simulink model "internal_cluster_fault"  (R2024b)
settings: Solver=VariableStepAuto  StartTime=0.0  StopTime=120  RelTol=1e-3
undefined symbols (not defined in the file): Ion, Lithium
libraries: spsIGBTDiodeLib x12, spsSeriesRLCBranchLib x4, spsBatteryLib x3, sps_lib x1
settings Model: Creator=Ranbir  LastModifiedBy=Ranbir

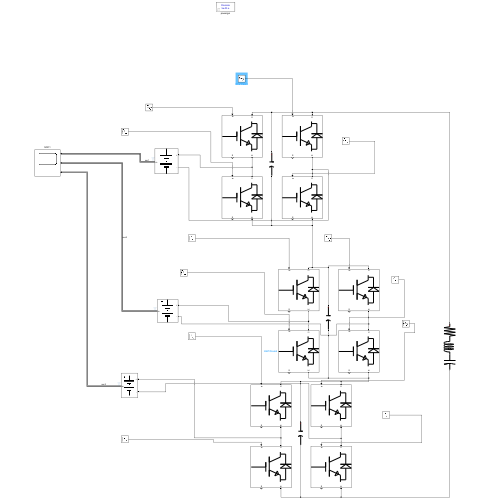
[thumbnail: Simulink's stored preview of the top-level diagram]
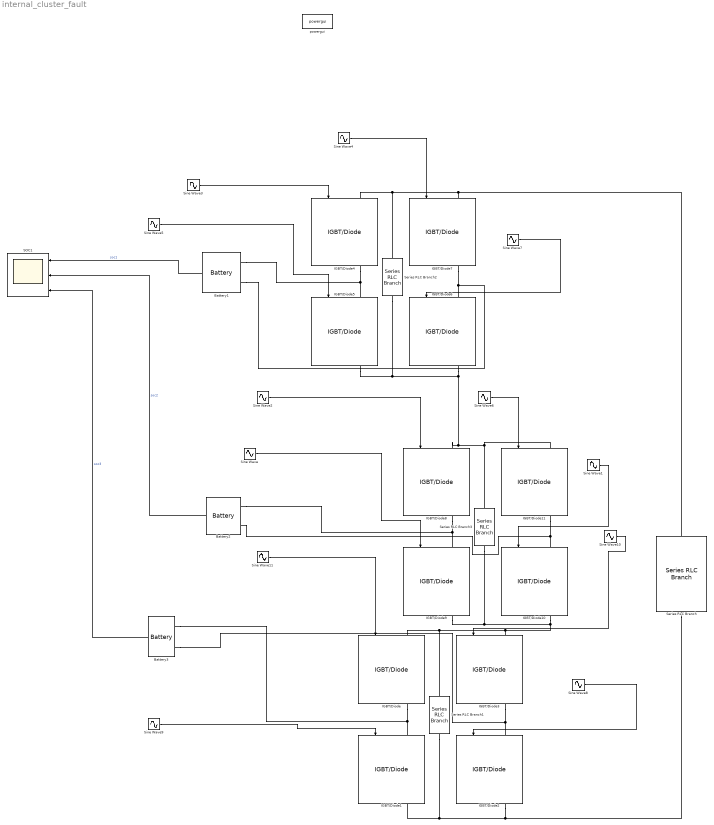
== system internal_cluster_fault ==
  Battery1 : spsBatteryLib/Battery  BatType=Lithium-Ion  NomV=7.2  NomQ=5.4  SOC=75  Batt_Tr=30  PresetModel=on  MaxQ=5.4  MinV=5.4  FullV=8.3807  Dis_rate=2.3478  R=0.013333  Normal_OP=4.8835  expZone="[7.7788      0.2653]"
  Battery2 : spsBatteryLib/Battery  BatType=Lithium-Ion  NomV=7.2  NomQ=5.4  SOC=95  Batt_Tr=30  PresetModel=on  MaxQ=5.4  MinV=5.4  FullV=8.3807  Dis_rate=2.3478  R=0.013333  Normal_OP=4.8835  expZone="[7.7788      0.2653]"
  Battery3 : spsBatteryLib/Battery  BatType=Lithium-Ion  NomV=7.2  NomQ=5.4  SOC=90  Batt_Tr=30  PresetModel=on  MaxQ=5.4  MinV=5.4  FullV=8.3807  Dis_rate=2.3478  R=0.013333  Normal_OP=4.8835  expZone="[7.7788      0.2653]"
  IGBT/Diode{,1..11} (12 alike) : spsIGBTDiodeLib/IGBT//Diode  Ron=1e-3  Rs=1e5  Cs=inf  Measurements=on
  SOC1 : Scope  NumInputPorts=3
  Series RLC Branch : spsSeriesRLCBranchLib/Series RLC Branch  LConnTagsString=__new0  RConnTagsString=__new0  BranchType=RLC  Resistance=1  Inductance=1e-3  SetiL0=off  InitialCurrent=0  Capacitance=1e-6  Setx0=off  InitialVoltage=0  Measurements=None
  Series RLC Branch1 : spsSeriesRLCBranchLib/Series RLC Branch  LConnTagsString=__new0  RConnTagsString=__new0  BranchType=C  Resistance=10  Inductance=1e-3  SetiL0=off  InitialCurrent=0  Capacitance=1e-6  Setx0=off  InitialVoltage=0  Measurements=Branch voltage and current
  Series RLC Branch2 : spsSeriesRLCBranchLib/Series RLC Branch  LConnTagsString=__new0  RConnTagsString=__new0  BranchType=C  Resistance=10  Inductance=1e-3  SetiL0=off  InitialCurrent=0  Capacitance=1e-6  Setx0=off  InitialVoltage=0  Measurements=Branch voltage and current
  Series RLC Branch3 : spsSeriesRLCBranchLib/Series RLC Branch  LConnTagsString=__new0  RConnTagsString=__new0  BranchType=C  Resistance=10  Inductance=1e-3  SetiL0=off  InitialCurrent=0  Capacitance=1e-6  Setx0=off  InitialVoltage=0  Measurements=Branch voltage and current
  Sine Wave{,1..3,5..11} (11 alike) : Sin  SampleTime=0
  Sine Wave4 : Sin  Bias=1  Frequency=2*pi*50  SampleTime=0
  powergui : sps_lib/powergui  Priority=1  SimulationMode=Discrete  SampleTime=50e-6  frequency=60  Iterations=50  frequencyindice=0  Pbase=100e6  ErrMax=1e-4  UnitsV=kV  UnitsW=MW  buscounter=0  FunctionMessages=off  echomessages=off  EnableUseOfTLC=off  CurrentSourceSwitches=off  DisableSnubberDevices=off  DisableRonSwitches=off  DisableVfSwitches=off  DisplayEquations=off  AutomaticDiscreteSolvers=off  SolverType=Tustin/Backward Euler (TBE)  Interpol=off  ExternalGateDelay=off  methode=off  Ts=100  x0status=blocks  SPID=on  SwTol=0  HookPort=off  NonlinearTolerance=1e-4  nMaxIteration=100  ContinueOnMaxIteration=off  RestoreLinks=warning  ResistiveCurrentMeasurement=off  Frange=[0:2:500]  Ylog=off  Xlog=on  ShowGrid=off  save=off  variable=ZData  structure=0  ZoomFFT=off  StartTime=0.0  cycles=1  DisplayStyle=1  fundamental=60  FreqAxis=off  MaxFrequency=1000  frequencyindicesteady=1  RmsSteady=1  display=off
  wires:
  Battery1/1 -> SOC1/1  "soc1"
  Battery2/1 -> SOC1/2  "soc2"
  Battery3/1 -> SOC1/3  "soc3"
  Sine Wave3/1 -> IGBT/Diode4/1
  Sine Wave4/1 -> IGBT/Diode7/1
  Sine Wave5/1 -> IGBT/Diode5/1
  Sine Wave1/1 -> IGBT/Diode10/1
  Sine Wave/1 -> IGBT/Diode9/1
  Sine Wave11/1 -> IGBT/Diode/1
  Sine Wave10/1 -> IGBT/Diode3/1
  Sine Wave6/1 -> IGBT/Diode11/1
  Sine Wave2/1 -> IGBT/Diode8/1
  Sine Wave7/1 -> IGBT/Diode6/1
  Sine Wave9/1 -> IGBT/Diode1/1
  Sine Wave8/1 -> IGBT/Diode2/1
  connections:
  IGBT/Diode4/LConn1 -- Series RLC Branch/LConn1 -- IGBT/Diode7/LConn1 -- Series RLC Branch2/LConn1
  IGBT/Diode4/RConn1 -- Battery1/LConn1 -- IGBT/Diode5/LConn1
  IGBT/Diode7/RConn1 -- Battery1/LConn2 -- IGBT/Diode6/LConn1
  IGBT/Diode8/LConn1 -- Series RLC Branch2/RConn1 -- IGBT/Diode5/RConn1 -- IGBT/Diode6/RConn1 -- IGBT/Diode11/LConn1 -- Series RLC Branch3/LConn1
  IGBT/Diode8/RConn1 -- Battery2/LConn1 -- IGBT/Diode9/LConn1
  IGBT/Diode11/RConn1 -- Battery2/LConn2 -- IGBT/Diode10/LConn1
  IGBT/Diode1/RConn1 -- Series RLC Branch/RConn1 -- IGBT/Diode2/RConn1 -- Series RLC Branch1/RConn1
  IGBT/Diode/LConn1 -- Series RLC Branch3/RConn1 -- IGBT/Diode9/RConn1 -- IGBT/Diode10/RConn1 -- IGBT/Diode3/LConn1 -- Series RLC Branch1/LConn1
  IGBT/Diode3/RConn1 -- Battery3/LConn2 -- IGBT/Diode2/LConn1
  IGBT/Diode/RConn1 -- Battery3/LConn1 -- IGBT/Diode1/LConn1
